simulink model "F_c_Linearizovana_staticka_karakteristika_20_80"  (R2016a)
settings: Solver=VariableStepAuto  StartTime=0.0  StopTime=800  RelTol=1e-3
libraries: simulink x2
settings Model: Creator=AmelT  LastModifiedBy=AmelT

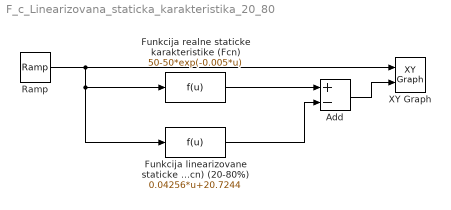
== system F_c_Linearizovana_staticka_karakteristika_20_80 ==
  Add : Sum  Inputs=+-
  Funkcija linearizovane staticke karakteristike (Fcn) (20-80%) : Fcn  Expr=0.04256*u+20.7244
  Funkcija realne staticke karakteristike (Fcn) : Fcn  Expr=50-50*exp(-0.005*u)
  Ramp : simulink/Sources/Ramp  slope=1  start=0  X0=0
  XY Graph : simulink/Sinks/XY Graph  xmin=0  xmax=800  ymin=-20  ymax=20  st=1
  wires:
  Ramp/1 -> XY Graph/1, Funkcija linearizovane staticke karakteristike (Fcn) (20-80%)/1, Funkcija realne staticke karakteristike (Fcn)/1
  Funkcija realne staticke karakteristike (Fcn)/1 -> Add/1
  Funkcija linearizovane staticke karakteristike (Fcn) (20-80%)/1 -> Add/2
  Add/1 -> XY Graph/2
